simulink model "PI_approx"  (R2020b)
settings: Solver=VariableStepAuto  StartTime=0.0  StopTime=10.0  RelTol=1e-3
undefined symbols (not defined in the file): T, T_i
settings Model: Creator=jasper  LastModifiedBy=jasper

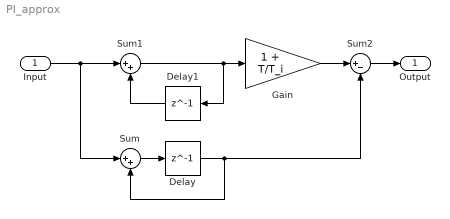
== system PI_approx ==
  Input : Inport
  Delay : Delay  DelayLength=1  SampleTime=T
  Delay1 : Delay  DelayLength=1  SampleTime=T
  Gain : Gain  Gain=1 + T/T_i
  Sum : Sum  Inputs=|++
  Sum1 : Sum  Inputs=|++
  Sum2 : Sum  Inputs=|+-
  Output : Outport
  wires:
  Sum/1 -> Delay/1
  Delay/1 -> Sum2/2, Sum/2
  Sum1/1 -> Gain/1, Delay1/1
  Delay1/1 -> Sum1/2
  Gain/1 -> Sum2/1
  Input/1 -> Sum/1, Sum1/1
  Sum2/1 -> Output/1
